simulink model "boeing747_lateral_control_simulink"  (R2023a)
settings: Solver=VariableStepAuto  StartTime=0.0  StopTime=10.0  RelTol=1e-3
undefined symbols (not defined in the file or in its folder): sys
settings Model: Creator=franc  LastModifiedBy=franc

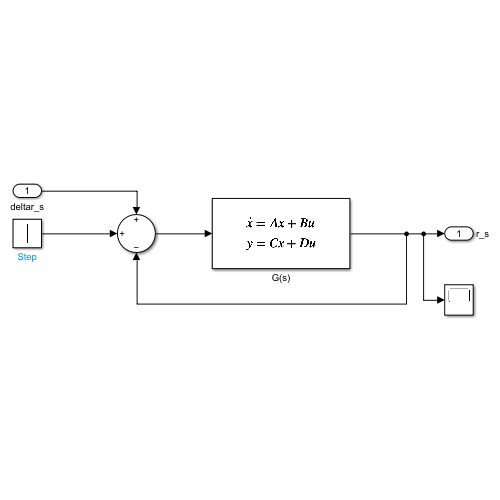
[thumbnail: Simulink's stored preview of the top-level diagram]
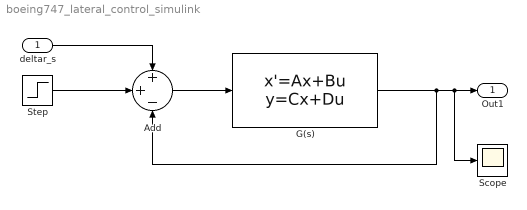
== system boeing747_lateral_control_simulink ==
  deltar_s : Inport
  Add : Sum  Inputs=++-
  G(s) : StateSpace  A=sys.A  B=sys.B  C=sys.C  D=sys.D  InitialCondition=0
  Scope : Scope
  Step : Step  SampleTime=0
  Out1 : Outport  SignalName=r_s
  wires:
  G(s)/1 -> Add/3, Scope/1, Out1/1
  deltar_s/1 -> Add/1
  Add/1 -> G(s)/1
  Step/1 -> Add/2
